simulink model "sensorMCUSlugsMKII"  (Simulink 6.6)
settings: Solver=FixedStepDiscrete  StartTime=0.0  StopTime=10.0  FixedStep=0.01  RelTol=1e-3
InitFcn:
  | mcuInit
values from neighbouring files (symbols this model uses):
  T = 0.01    [initGPS.m]    (also in mcuInit.m)
undefined symbols (not defined in the file or in its folder): baroMeanTemp, baroOffset, baroScale, baroTempK, baseHeight, baseTemp, cubeAccelGain, cubeGyroGain, gaind, getCubeData, getGpsMainData, getMag, hil_getEuler, hil_getRates, hil_getRawRead, hil_getVned, hil_getXYZ, hilRead, lapseRate, logData, magMeanTemp, magOffset, magScale, magTempK, pitotOffset, pitotScale, polesd, powerOffset, powerScale, protParseDecode, sensorMCUInit, spiSend, tempOffset, tempScale, u1, u2, updateAirData, updateAttitude, updateBias, updateDiagnosticFl, updateDiagnosticSh, updateLoadData, updatePilotConsole, updatePosition, updateRawADCData, updateTimeStamp, y1, zerosd
libraries: dsPICdrivers x37, simulink x3, aerolibconvert2 x1
(part 2 of 2)

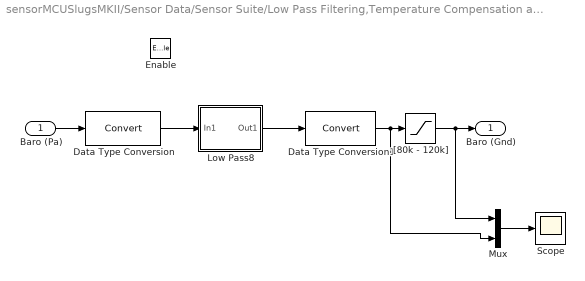
== system sensorMCUSlugsMKII/Sensor Data/Sensor Suite/Low Pass Filtering,Temperature Compensation and Calibration/Baro Altimeter/Initial Baro Bias ==
  Baro (Pa) : Inport
  Enable : EnablePort
  Data Type Conversion : DataTypeConversion  OutDataTypeMode=double
  Data Type Conversion1 : DataTypeConversion  OutDataTypeMode=single
  Low Pass8 : Subsystem  mask(DiscretizedZeroPole){Zeros=[], Poles=[-3], Gain=3, AbsTol=auto, SampleTime=.01, method=tustin, Wc=1}
      mask prompts: Zeros "Zeros (enter in s-main:)"; Poles "Poles (enter in s-domain:)"; Gain "Gain (enter in s-domain:)"; AbsTol "Absolute tolerance:"; SampleTime "Sample time:"; Wc "Critical Frequency (Hz):"
      mask help: Continuous mask uses c2d to transform parameters onto the Discrete Zero-Pole block inside.
      mask init: same as sensorMCUSlugsMKII/Sensor Data/Sensor Suite/Low Pass Filtering,Temperature Compensation and Calibration/Low Pass1
      mask StyleString: edit,edit,edit,edit,edit,popup(zoh|foh|tustin|prewarp|matched),edit
      mask CallbackString: |||||hidecrit|
      mask Display:
      | droots(zeross,poless,gainss)
      | text( 0.5, 1.0, method, 'verticalAlignment','top')
  Mux : Mux  Inputs=2
  Scope : Scope
      settings: SaveName=ScopeData8
  "[80k - 120k]" : Saturate  UpperLimit=120000  LowerLimit=80000
  Baro (Gnd) : Outport
  wires:
  Baro (Pa)/1 -> Data Type Conversion/1
  Low Pass8/1(Out1) -> Data Type Conversion1/1
  Data Type Conversion/1 -> Low Pass8/1(In1)
  Data Type Conversion1/1 -> Mux/2, "[80k - 120k]"/1
  Mux/1 -> Scope/1
  "[80k - 120k]"/1 -> Baro (Gnd)/1, Mux/1

== system sensorMCUSlugsMKII/Sensor Data/Sensor Suite/Low Pass Filtering,Temperature Compensation and Calibration/Baro Altimeter/Zero Out Height ==
  Base Height : Inport
  Computed Height : Inport  Port=2
  Enable : EnablePort
  Integer Delay : simulink/Discrete/Integer Delay  vinit=0  samptime=.01  NumDelays=1
  Sum : Sum  Inputs=|+-  OutDataTypeMode=single
  Height Offset : Outport
  wires:
  Computed Height/1 -> Integer Delay/1
  Sum/1 -> Height Offset/1
  Integer Delay/1 -> Sum/2
  Base Height/1 -> Sum/1

== system sensorMCUSlugsMKII/Sensor Data/Sensor Suite/Low Pass Filtering,Temperature Compensation and Calibration/Baro Altimeter/Initial Baro Bias/Low Pass8 ==
  In1 : Inport
  Discrete Zero-Pole : DiscreteZeroPole  Zeros=zerosd  Poles=polesd  Gain=gaind  SampleTime=SampleTime
  Out1 : Outport
  wires:
  In1/1 -> Discrete Zero-Pole/1
  Discrete Zero-Pole/1 -> Out1/1

== matlab function Sensor Data/Sensor Suite/myMux Fun ==
  data: u1 input inherited; y output inherited; u2 input inherited; u3 input inherited
function y = myMux3(u1, u2, u3)
% This block supports an embeddable subset of the MATLAB language.
% See the help menu for details. 

y = [u1(1); u2(1); u3(1)];

== matlab function myMux Fun1 ==
  data: u1 input inherited; y output inherited; u2 input inherited; u3 input inherited
function y = myMux3(u1, u2, u3)
% This block supports an embeddable subset of the MATLAB language.
% See the help menu for details. 

y = [u1(1); u2(1); u3(1)];

== matlab function myMux Fun5 ==
  data: u1 input inherited; y output inherited; u2 input inherited; u3 input inherited
function y = myMux3(u1, u2, u3)
% This block supports an embeddable subset of the MATLAB language.
% See the help menu for details. 

y = [u1(1); u2(1); u3(1)];

== matlab function myMux Fun4 ==
  data: u1 input inherited; y output inherited; u2 input inherited
function y = myMux(u1, u2)
% This block supports an embeddable subset of the MATLAB language.
% See the help menu for details. 

y = [u1(1:3); u2(1:3)];

== matlab function myMux Fun3 ==
  data: u1 input inherited; y output inherited; u2 input inherited
function y = myMux(u1, u2)
% This block supports an embeddable subset of the MATLAB language.
% See the help menu for details. 

y = [u1(1:3); u2(1:3)];

== matlab function Sensor Data/Sensor Suite/Low Pass Filtering,Temperature Compensation and Calibration/3D Filter/myMux Fun1 ==
  data: u1 input inherited; y output inherited; u2 input inherited; u3 input inherited
function y = myMux(u1, u2, u3)
% This block supports an embeddable subset of the MATLAB language.
% See the help menu for details. 

y = [u1(1); u2(1); u3(1)];

== matlab function Sensor Data/Sensor Suite/Low Pass Filtering,Temperature Compensation and Calibration/Baro Altimeter/Enables/Disables the Computation of initial Baro Bias ==
  data: tOut output inherited
function tOut = getTIni

persistent aveCount;
persistent tIni;

if isempty(aveCount)
    aveCount =1;
    tIni = 1;
end;

if aveCount < 500
    aveCount = aveCount + 1;
end

if aveCount == 500
    tIni =0;
    aveCount = aveCount + 1;
end

tOut = tIni;

%if aveCount > 500
%    tIni = 0;
%end

% if isempty(aveCount)
%     aveCount =1;
%     initBias = [0.0 0.0 0.0]';
% end;
%     
% if (aveCount<10)
%     initBias = initBias+ Raw;
%     bias = initBias/aveCount;
%     aveCount = aveCount +1;
% end;
% 
% if (aveCount == 10)
%     initBias = initBias/(aveCount-1);
%     aveCount = 100;
% end;
% 
% if (aveCount == 100)
%     bias = initBias;
% end;

== matlab function myMux Fun2 ==
  data: u1 input inherited; y output inherited; u2 input inherited
function y = myMux(u1, u2)
% This block supports an embeddable subset of the MATLAB language.
% See the help menu for details. 

y = [u1(1:3); u2(1:3)];

== matlab function Control Surface Input/myMux Fun5 ==
  data: u1 input inherited; y output inherited; u2 input inherited; u3 input inherited; u4 input inherited; u5 input inherited
function y = myMux(u1, u2, u3, u4, u5)
% This block supports an embeddable subset of the MATLAB language.
% See the help menu for details. 

y = [u1(1); u2(1); u3(1); u4(1); u5(1)];

== matlab function Sensor Data/Sensor Suite/If no HIL then Read all the Sensors/myMux Fun4 ==
  data: u1 input inherited; y output inherited; u2 input inherited; u3 input inherited; u4 input inherited; u5 input inherited; u6 input inherited; u7 input inherited; u8 input inherited; u9 input inherited; u10 input inherited; u11 input inherited; u12 input inherited; u13 input inherited
function y = sensMux(u1, u2,u3,u4,u5,u6,u7,u8, u9, u10, u11, u12, u13)
% This block supports an embeddable subset of the MATLAB language.
% See the help menu for details. 

y = [u1(1); u2(1); u3(1); u4(1); u5(1); u6(1); u7(1); u8(1); u9(1); u10(1); u11(1); u12(1); u13(1)];

== matlab function Sensor Data/Sensor Suite/If no HIL then Read all the Sensors/myMux Fun ==
  data: u1 input inherited; y output inherited; u2 input inherited; u3 input inherited; u4 input inherited
function y = myMux(u1, u2, u3, u4)
% This block supports an embeddable subset of the MATLAB language.
% See the help menu for details. 

y = [u1(1); u2(1); u3(1); u4(1)];
